simulink model "Incubadora"  (R2025b)
settings: Solver=VariableStepAuto  StartTime=0.0  StopTime=1000  RelTol=1e-3
settings Model: SimulationMode=rapid-accelerator  ExtModeTrigDuration=100
settings GRTTargetCC: RTWCAPISignals=on  RTWCAPIParams=on

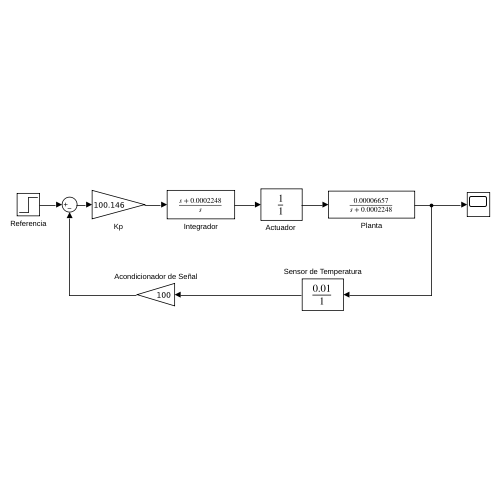
[thumbnail: Simulink's stored preview of the top-level diagram]
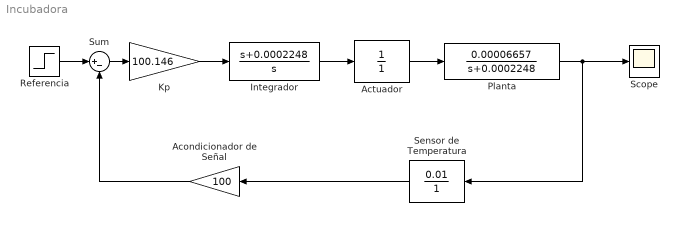
== system Incubadora ==
  Acondicionador de Señal : Gain  Gain=100
  "Actuador " : TransferFcn  Denominator=[1 ]  ContinuousStateAttributes=Actuador
  Integrador : TransferFcn  Numerator=[1 0.0002248]  Denominator=[1 0]
  Kp : Gain  Gain=100.146
  Planta : TransferFcn  Numerator=[0.00006657]  Denominator=[1 0.0002248]
  Referencia : Step  Time=100000  After=37.7  SampleTime=0
  Scope : Scope
      settings: ActiveDisplayYMinimum=-0.2563917404303378  ActiveDisplayYMaximum=2.3075256638730406
  Sensor de Temperatura : TransferFcn  Numerator=[0.01]  Denominator=[1 ]
  Sum : Sum  Inputs=|+-
  wires:
  "Actuador "/1 -> Planta/1
  Sensor de Temperatura/1 -> Acondicionador de Señal/1
  Kp/1 -> Integrador/1
  Sum/1 -> Kp/1
  Planta/1 -> Scope/1, Sensor de Temperatura/1
  Acondicionador de Señal/1 -> Sum/2
  Referencia/1 -> Sum/1
  Integrador/1 -> "Actuador "/1
